simulink model "MPC_deploy"  (R2020b)
settings: Solver=FixedStepAuto  StartTime=0.0  StopTime=24*60*60  FixedStep=60  RelTol=1e-7  EnableMultiTasking=on
libraries: embdlinuxlib x10, mpclib x1
settings Model: Creator=enzlp  LastModifiedBy=Triphase_Setup
settings SolverCC: AlgebraicLoopSolver=LineSearch  PositivePriorityOrder=on
settings DataIOCC: SaveFormat=Array  ReturnWorkspaceOutputs=off
settings OptimizationCC: EnhancedBackFolding=on  PassReuseOutputArgsAs=Individual arguments  ZeroExternalMemoryAtStartup=off  ZeroInternalMemoryAtStartup=off  MaxStackSize=64  OptimizeBlockOrder=speed  DifferentSizesBufferReuse=on  OptimizationCustomize=off  EfficientTunableParamExpr=on
settings DebuggingCC: ParameterTunabilityLossMsg=error
settings HardwareCC: ProdBitPerPointer=32  ProdBitPerSizeT=32  ProdBitPerPtrDiffT=32  ProdLargestAtomicInteger=Long  ProdLargestAtomicFloat=Double  ProdWordSize=32  ProdLongLongMode=on  ProdHWDeviceType=ARM Compatible->ARM Cortex
settings RTWCC: Description=Embedded Coder  SystemTargetFile=ert.tlc  HardwareBoard=Raspberry Pi  TLCOptions="-aInlineSetEventsForThisBaseRateFcn=TLC_FALSE -aSuppressMultiTaskScheduler=TLC_FALSE  -aRateBasedStepFcn=0"  TemplateMakefile=ert_default_tmf  Toolchain=GNU GCC Raspberry Pi  BuildConfiguration=Faster Runs
settings CodeAppCC: ForceParamTrailComments=on  IgnoreCustomStorageClasses=off  OperatorAnnotations=on  SimulinkDataObjDesc=on  SFDataObjDesc=on  InsertBlockDesc=on
settings ERTTargetCC: SupportVariableSizeSignals=on  ExtModeTransport=2  ExtModeMexFile=ext_xcp  ExtModeIntrfLevel=Level2 - Open

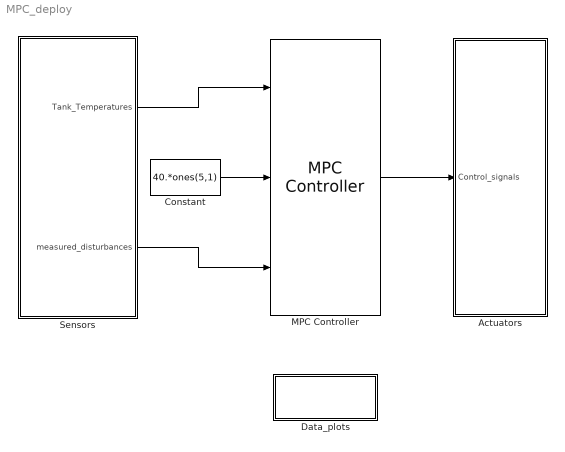
== system MPC_deploy ==
  Actuators : Subsystem
  Constant : Constant  Value=40.*ones(5,1)
  Data_plots : Subsystem
  MPC Controller : mpclib/MPC Controller  SCDEnableBlockLinearizationSpecification=on  mpcobj=mpc1  is_multiple=0  enable_value=0  return_u0=off  updateMPCinCallerWorkspace=on  md_inport=on  mv_inport=off  uref_inport=off  return_cost=off  return_mvseq=off  return_qpstatus=off  return_xseq=off  return_state=off  return_ovseq=off  state_inport=off  umin_inport=off  umax_inport=off  ymin_inport=off  ymax_inport=off  cc_inport=off  ywt_inport=off  uwt_inport=off  duwt_inport=off  rhoeps_inport=off  pm_inport=off  MaximumP=10  HorizonChoice=FixedHorizon  n_ts=60  n_p=10  n_mv=2  n_md=3  n_ud=0  n_mo=5  n_uo=0  BlockDataType=double  SampleTimeInherited=off  switch_inport=off
  Sensors : Subsystem
  wires:
  MPC Controller/1 -> Actuators/1(Control_signals)
  Sensors/1(Tank_Temperatures) -> MPC Controller/1
  Sensors/2(measured_disturbances) -> MPC Controller/3
  Constant/1 -> MPC Controller/2

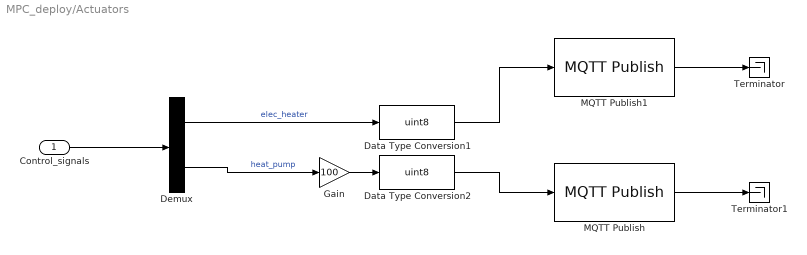
== system MPC_deploy/Actuators ==
  Control_signals : Inport
  Data Type Conversion1 : DataTypeConversion  OutDataTypeStr=uint8
  Data Type Conversion2 : DataTypeConversion  OutDataTypeStr=uint8
  Demux : Demux  Outputs=2
  Gain : Gain  Gain=100
  MQTT Publish : embdlinuxlib/MQTT Publish  Topic=valve2  QoS=0  RetainMsg=off
      settings: SourceProductBaseCode=SC_BEAGLEBONE_BLUE,NVIDIA,RASPPI
  MQTT Publish1 : embdlinuxlib/MQTT Publish  Topic=valve1  QoS=0  RetainMsg=off
      settings: SourceProductBaseCode=SC_BEAGLEBONE_BLUE,NVIDIA,RASPPI
  Terminator : Terminator
  Terminator1 : Terminator
  wires:
  Control_signals/1 -> Demux/1
  Data Type Conversion1/1 -> MQTT Publish1/1
  MQTT Publish1/1 -> Terminator/1
  Demux/1 -> Data Type Conversion1/1  "elec_heater"
  Demux/2 -> Gain/1  "heat_pump"
  Data Type Conversion2/1 -> MQTT Publish/1
  Gain/1 -> Data Type Conversion2/1
  MQTT Publish/1 -> Terminator1/1

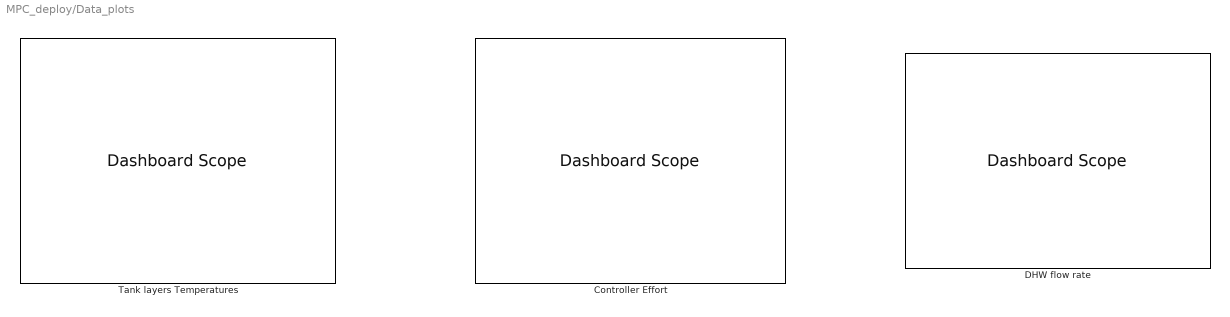
== system MPC_deploy/Data_plots ==
  Controller Effort : DashboardScope
  DHW flow rate : DashboardScope
  Tank layers Temperatures : DashboardScope

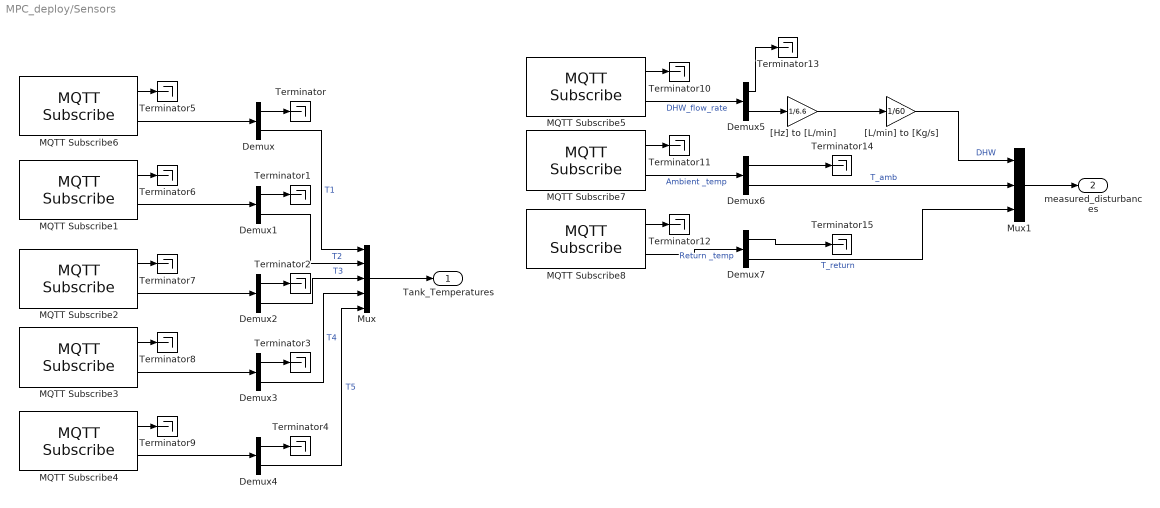
== system MPC_deploy/Sensors ==
  Demux{,1..7} (8 alike) : Demux  Outputs=2
  MQTT Subscribe1 : embdlinuxlib/MQTT Subscribe  Topic=temp2  QoS=0  MessageLength=2  SampleTime=1
      settings: SourceProductBaseCode=SC_BEAGLEBONE_BLUE,NVIDIA,RASPPI
  MQTT Subscribe2 : embdlinuxlib/MQTT Subscribe  Topic=temp3  QoS=0  MessageLength=2  SampleTime=1
      settings: SourceProductBaseCode=SC_BEAGLEBONE_BLUE,NVIDIA,RASPPI
  MQTT Subscribe3 : embdlinuxlib/MQTT Subscribe  Topic=temp4  QoS=0  MessageLength=2  SampleTime=1
      settings: SourceProductBaseCode=SC_BEAGLEBONE_BLUE,NVIDIA,RASPPI
  MQTT Subscribe4 : embdlinuxlib/MQTT Subscribe  Topic=temp5  QoS=0  MessageLength=2  SampleTime=1
      settings: SourceProductBaseCode=SC_BEAGLEBONE_BLUE,NVIDIA,RASPPI
  MQTT Subscribe5 : embdlinuxlib/MQTT Subscribe  Topic=flow1  QoS=0  MessageLength=2  SampleTime=1
      settings: SourceProductBaseCode=SC_BEAGLEBONE_BLUE,NVIDIA,RASPPI
  MQTT Subscribe6 : embdlinuxlib/MQTT Subscribe  Topic=temp1  QoS=0  MessageLength=2  SampleTime=1
      settings: SourceProductBaseCode=SC_BEAGLEBONE_BLUE,NVIDIA,RASPPI
  MQTT Subscribe7 : embdlinuxlib/MQTT Subscribe  Topic=temp6  QoS=0  MessageLength=2  SampleTime=1
      settings: SourceProductBaseCode=SC_BEAGLEBONE_BLUE,NVIDIA,RASPPI
  MQTT Subscribe8 : embdlinuxlib/MQTT Subscribe  Topic=temp7  QoS=0  MessageLength=2  SampleTime=1
      settings: SourceProductBaseCode=SC_BEAGLEBONE_BLUE,NVIDIA,RASPPI
  Mux : Mux  Inputs=5
  Mux1 : Mux  Inputs=3
  Terminator{,1..15} (16 alike) : Terminator
  "[Hz] to [L/min]" : Gain  Gain=1/6.6
  "[L/min] to [Kg/s]" : Gain  Gain=1/60
  Tank_Temperatures : Outport
  measured_disturbances : Outport  Port=2
  wires:
  MQTT Subscribe6/2 -> Demux/1
  Demux/1 -> Terminator/1
  MQTT Subscribe1/2 -> Demux1/1
  Demux1/1 -> Terminator1/1
  MQTT Subscribe2/2 -> Demux2/1
  Demux2/1 -> Terminator2/1
  Demux3/1 -> Terminator3/1
  MQTT Subscribe3/2 -> Demux3/1
  Demux4/1 -> Terminator4/1
  MQTT Subscribe4/2 -> Demux4/1
  Mux/1 -> Tank_Temperatures/1
  Demux/2 -> Mux/1  "T1"
  Demux1/2 -> Mux/2  "T2"
  Demux2/2 -> Mux/3  "T3"
  Demux3/2 -> Mux/4  "T4"
  Demux4/2 -> Mux/5  "T5"
  MQTT Subscribe6/1 -> Terminator5/1
  MQTT Subscribe1/1 -> Terminator6/1
  MQTT Subscribe2/1 -> Terminator7/1
  MQTT Subscribe3/1 -> Terminator8/1
  MQTT Subscribe4/1 -> Terminator9/1
  "[L/min] to [Kg/s]"/1 -> Mux1/1  "DHW"
  MQTT Subscribe5/1 -> Terminator10/1
  MQTT Subscribe5/2 -> Demux5/1  "DHW_flow_rate"
  Demux5/1 -> Terminator13/1
  MQTT Subscribe7/1 -> Terminator11/1
  MQTT Subscribe7/2 -> Demux6/1  "Ambient _temp"
  MQTT Subscribe8/1 -> Terminator12/1
  Demux6/1 -> Terminator14/1
  MQTT Subscribe8/2 -> Demux7/1  "Return _temp"
  Demux7/1 -> Terminator15/1
  Demux6/2 -> Mux1/2  "T_amb"
  Demux7/2 -> Mux1/3  "T_return"
  Mux1/1 -> measured_disturbances/1
  Demux5/2 -> "[Hz] to [L/min]"/1
  "[Hz] to [L/min]"/1 -> "[L/min] to [Kg/s]"/1
